simulink model "teleoperation_2017b"  (R2018a)
settings: Solver=ode45  StartTime=0.0  StopTime=10  FixedStep=0.001  RelTol=1e-3
values from neighbouring files (symbols this model uses):
  B_e = 0.01    [Teleop.m]    (also in simulinkTeleop.m)
  B_h = 4.0    (= 4)    [Teleop.m]    (also in simulinkTeleop.m = 0.4)
  B_v = 0.15    [Teleop.m]    (also in simulinkTeleop.m)
  J_m = 0.0005    [Teleop.m]    (also in simulinkTeleop.m)
  J_s = 0.0005    [Teleop.m]    (also in simulinkTeleop.m)
  J_v = 0.0    (= 0)    [Teleop.m]    (also in simulinkTeleop.m)
  K_h = 200.0    (= 200)    [Teleop.m]    (also in simulinkTeleop.m = 20)
  K_v = 100.0    (= 100)    [Teleop.m]    (also in simulinkTeleop.m)
libraries: cstblocks x5, simulink x1
settings Model: Creator=blue_orangotan  LastModifiedBy=blue_orangotan
settings CodeAppCC: StateflowObjectComments=on

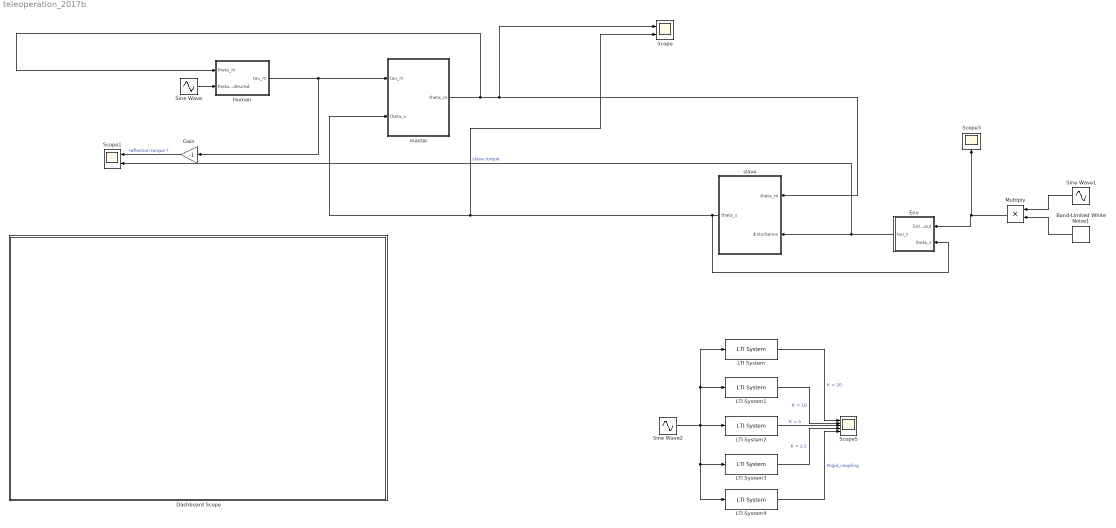
== system teleoperation_2017b ==
  Band-Limited White Noise1 : simulink/Sources/Band-Limited White Noise  Cov=0.001  Ts=0.001  seed=[12345]
  Dashboard Scope : Subsystem  DialogController=hmiCreateDDGDialog  IsWebBlock=on  mask(MWDashboardBlock){webBlockId=d953983e-eab8-4310-ba24-9145e9f5b59c, webBlockType=sdiscope, ShowInitialText=on, HMISrcModelName=teleoperation_2017b}
      mask prompts: webBlockId "WebBlock Id"; webBlockType "WebBlock Type"; HMISrcModelName "Source Model"
      mask help: SimulinkHMI:dialogs:HMIScopeDialogDesc
      mask Help: helpview([docroot '/mapfiles/simulink.map'], 'hmi_scope')
      mask Display:
      | if strcmp(get_param(bdroot(gcb),'BlockDiagramType'), 'library')
      |     image([(matlabroot) '/toolbox/simulink/hmi/icons/DashboardScope.png']);
      | end
  Env : Subsystem
  Gain : Gain  Gain=-1
  Human : Subsystem
  LTI System : cstblocks/LTI System  sys=set_1  IC=[]
  LTI System1 : cstblocks/LTI System  sys=set_2  IC=[]
  LTI System2 : cstblocks/LTI System  sys=set_3  IC=[]
  LTI System3 : cstblocks/LTI System  sys=set_4  IC=[]
  LTI System4 : cstblocks/LTI System  sys=rigid  IC=[]
  Multiply : Product
  Scope : Scope  NumInputPorts=2
  Scope1 : Scope  NumInputPorts=2
  Scope3 : Scope
  Scope5 : Scope  NumInputPorts=5
  Sine Wave : Sin  Amplitude=0.18  Frequency=0.11*(6.28)  SampleTime=0
  Sine Wave1 : Sin  Amplitude=0.1  Frequency=100*(6.28)  SampleTime=0
  Sine Wave2 : Sin  Amplitude=0.1  Frequency=50*(6.28)  SampleTime=0
  master : Subsystem
  "slave " : Subsystem
  wires:
  master/1(theta_m) -> "slave "/1("theta_m "), Scope/1, Human/1(theta_m)
  "slave "/1(theta_s) -> Scope/2, master/2(theta_s), Env/2(theta_s)
  Env/1("tau_s ") -> Scope1/2, "slave "/2(disturbance)  "slave torque"
  Sine Wave/1 -> Human/2(theta_desired)
  Human/1(tau_m) -> Gain/1, master/1(tau_m)
  Sine Wave2/1 -> LTI System4/1, LTI System3/1, LTI System2/1, LTI System1/1, LTI System/1
  LTI System/1 -> Scope5/1  "K = 20"
  LTI System1/1 -> Scope5/2  "K = 10"
  LTI System2/1 -> Scope5/3  "K = 5"
  LTI System3/1 -> Scope5/4  "K = 2.5"
  LTI System4/1 -> Scope5/5  "Rigid_coupling"
  Gain/1 -> Scope1/1  "reflection torque ?"
  Sine Wave1/1 -> Multiply/1
  Band-Limited White Noise1/1 -> Multiply/2
  Multiply/1 -> Env/1(External_input), Scope3/1

== system teleoperation_2017b/Dashboard Scope ==

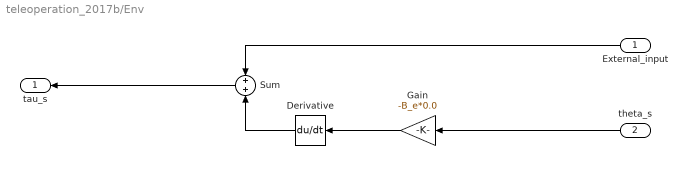
== system teleoperation_2017b/Env ==
  External_input : Inport
  theta_s : Inport  Port=2
  Derivative : Derivative  CoefficientInTFapproximation=0
  Gain : Gain  Gain=-B_e*0.0
  Sum : Sum
  "tau_s " : Outport
  wires:
  External_input/1 -> Sum/1
  theta_s/1 -> Gain/1
  Gain/1 -> Derivative/1
  Derivative/1 -> Sum/2
  Sum/1 -> "tau_s "/1

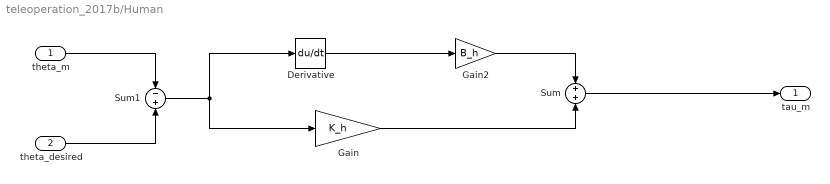
== system teleoperation_2017b/Human ==
  theta_m : Inport
  theta_desired : Inport  Port=2
  Derivative : Derivative  CoefficientInTFapproximation=0
  Gain : Gain  Gain=K_h
  Gain2 : Gain  Gain=B_h
  Sum : Sum  Inputs=+|+
  Sum1 : Sum  Inputs=-|+
  tau_m : Outport
  wires:
  Derivative/1 -> Gain2/1
  theta_m/1 -> Sum1/1
  theta_desired/1 -> Sum1/2
  Sum1/1 -> Derivative/1, Gain/1
  Gain2/1 -> Sum/1
  Gain/1 -> Sum/2
  Sum/1 -> tau_m/1

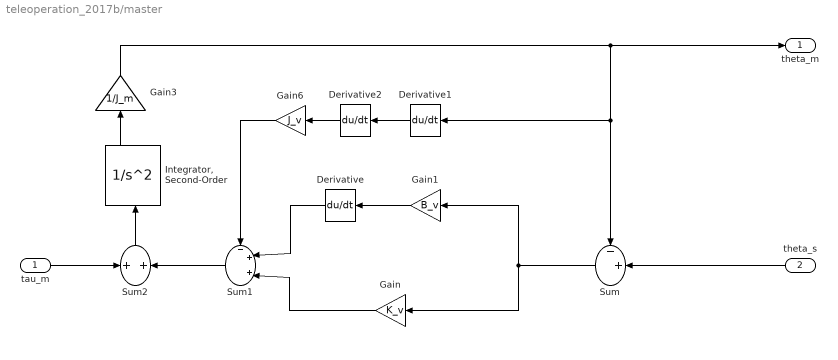
== system teleoperation_2017b/master ==
  tau_m : Inport
  theta_s : Inport  Port=2
  Derivative : Derivative  CoefficientInTFapproximation=0
  Derivative1 : Derivative  CoefficientInTFapproximation=0
  Derivative2 : Derivative  CoefficientInTFapproximation=0
  Gain : Gain  Gain=K_v
  Gain1 : Gain  Gain=B_v
  Gain3 : Gain  Gain=1/J_m
  Gain6 : Gain  Gain=J_v
  "Integrator, Second-Order" : SecondOrderIntegrator  ICX=0
  Sum : Sum  Inputs=-+|
  Sum1 : Sum  Inputs=-++|
  Sum2 : Sum  Inputs=+|+
  theta_m : Outport
  wires:
  Derivative1/1 -> Derivative2/1
  "Integrator, Second-Order"/1 -> Gain3/1
  theta_s/1 -> Sum/2
  Gain/1 -> Sum1/3
  Sum/1 -> Gain/1, Gain1/1
  Sum1/1 -> Sum2/2
  Derivative2/1 -> Gain6/1
  Derivative/1 -> Sum1/2
  Gain6/1 -> Sum1/1
  Gain1/1 -> Derivative/1
  Sum2/1 -> "Integrator, Second-Order"/1
  tau_m/1 -> Sum2/1
  Gain3/1 -> theta_m/1, Derivative1/1, Sum/1

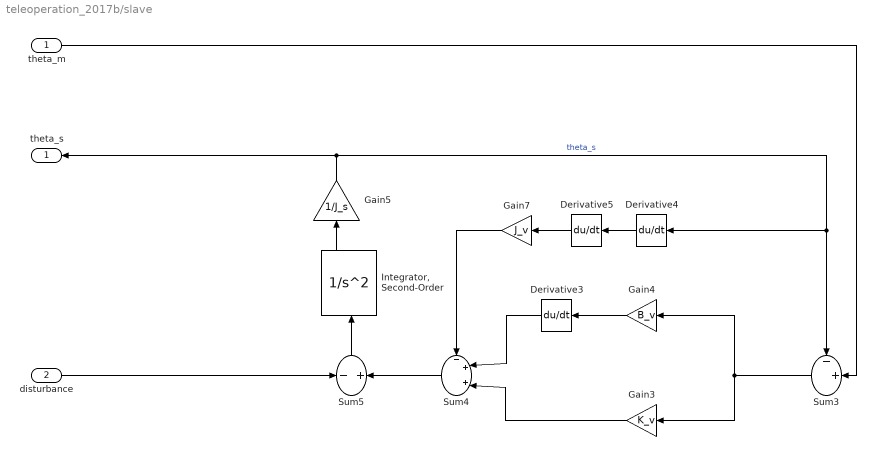
== system teleoperation_2017b/slave  ==
  "theta_m " : Inport
  disturbance : Inport  Port=2
  Derivative3 : Derivative  CoefficientInTFapproximation=0
  Derivative4 : Derivative  CoefficientInTFapproximation=0
  Derivative5 : Derivative  CoefficientInTFapproximation=0
  Gain3 : Gain  Gain=K_v
  Gain4 : Gain  Gain=B_v
  Gain5 : Gain  Gain=1/J_s
  Gain7 : Gain  Gain=J_v
  "Integrator, Second-Order" : SecondOrderIntegrator  ICX=0
  Sum3 : Sum  Inputs=-+|
  Sum4 : Sum  Inputs=-++|
  Sum5 : Sum  Inputs=-|+
  theta_s : Outport
  wires:
  Sum5/1 -> "Integrator, Second-Order"/1
  Gain7/1 -> Sum4/1
  "Integrator, Second-Order"/1 -> Gain5/1
  Derivative5/1 -> Gain7/1
  Sum4/1 -> Sum5/2
  Derivative3/1 -> Sum4/2
  Gain4/1 -> Derivative3/1
  Gain5/1 -> Derivative4/1, Sum3/1, theta_s/1  "theta_s"
  Gain3/1 -> Sum4/3
  "theta_m "/1 -> Sum3/2
  Sum3/1 -> Gain3/1, Gain4/1
  Derivative4/1 -> Derivative5/1
  disturbance/1 -> Sum5/1
